simulink model "hinfSL"  (R2022b)
settings: Solver=VariableStepAuto  StartTime=0.0  StopTime=50  RelTol=1e-3
undefined symbols (not defined in the file or in its folder): ang_Lin, G, K_hinf
libraries: simulink x1
settings Model: Creator=andre  LastModifiedBy=amoralesma
settings SolverCC: AlgebraicLoopSolver=TrustRegion
settings DebuggingCC: UnconnectedInputMsg=warning  UnconnectedOutputMsg=warning  UnconnectedLineMsg=warning  SFMachineParentedDataDiag=warning
settings ModelReferenceCC: EnableRefExpFcnMdlSchedulingChecks=on
settings RTWCC: DLArmComputeVersion=19.05

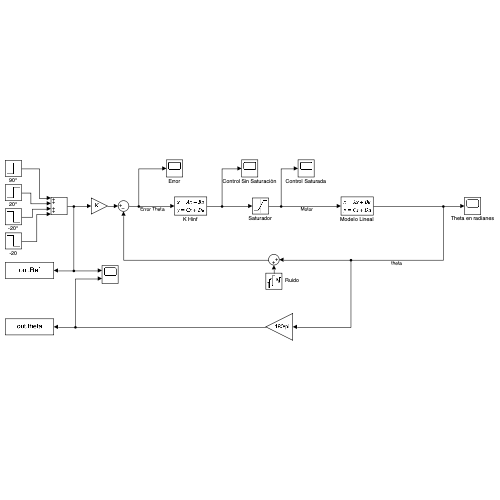
[thumbnail: Simulink's stored preview of the top-level diagram]
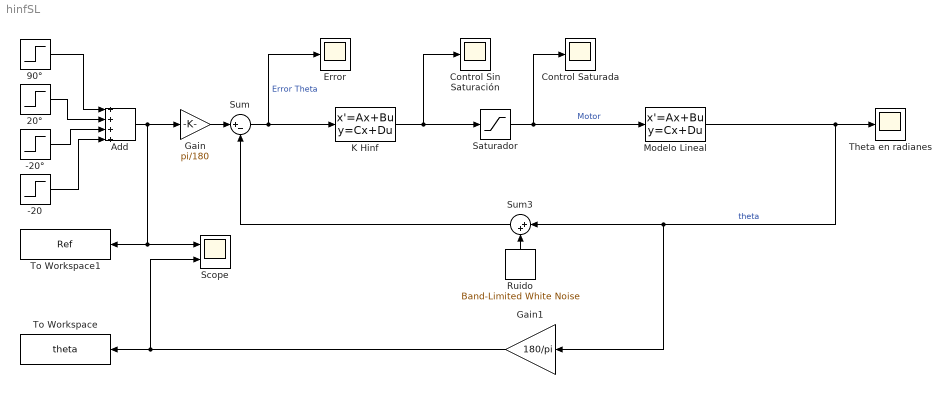
== system hinfSL ==
  -20 : Step  Time=30  After=-10  SampleTime=0
  -20° : Step  Time=20  After=-20  SampleTime=0
  20° : Step  Time=10  After=20  SampleTime=0
  90° : Step  Time=0  After=90  SampleTime=0
  Add : Sum  Inputs=++++
  Control Saturada : Scope
  Control Sin Saturación : Scope
  Error : Scope
  Gain : Gain  Gain=pi/180
  Gain1 : Gain  Gain=180/pi
  K Hinf : StateSpace  A=K_hinf.A  B=K_hinf.B  C=K_hinf.C  D=K_hinf.D  InitialCondition=0
  Modelo Lineal : StateSpace  A=G.A  B=G.B  C=G.C  D=G.D  InitialCondition=ang_Lin*(pi/180)
  Ruido : simulink/Sources/Band-Limited White Noise  Cov=[0.0001]  Ts=0.1  seed=[23341]
  Saturador : Saturate  UpperLimit=100  LowerLimit=0
  Scope : Scope  NumInputPorts=2
  Sum : Sum  Inputs=|+-
  Sum3 : Sum  Inputs=|++
  Theta en radianes : Scope
  To Workspace : ToWorkspace  VariableName=theta  SaveFormat=Timeseries  SampleTime=-1
  To Workspace1 : ToWorkspace  VariableName=Ref  SaveFormat=Timeseries  SampleTime=-1
  wires:
  Sum/1 -> Error/1, K Hinf/1  "Error Theta"
  90°/1 -> Add/1
  20°/1 -> Add/2
  Sum3/1 -> Sum/2
  Add/1 -> Gain/1, To Workspace1/1, Scope/1
  K Hinf/1 -> Control Sin Saturación/1, Saturador/1
  -20/1 -> Add/4
  Ruido/1 -> Sum3/2
  Modelo Lineal/1 -> Sum3/1, Gain1/1, Theta en radianes/1  "theta"
  -20°/1 -> Add/3
  Saturador/1 -> Control Saturada/1, Modelo Lineal/1  "Motor"
  Gain/1 -> Sum/1
  Gain1/1 -> To Workspace/1, Scope/2
